simulink model "war_pocz"  (R2014a)
settings: Solver=ode45  StartTime=0.0  StopTime=1  MaxStep=0.5  RelTol=1e-3
values from neighbouring files (symbols this model uses):
  A = [-Kcg1-Kcs-Kcw1 Kcg1 Kcs 0 0 0 ... (first row only)    [blok.m]
  B = [Kcw1 0 ... (first row only)    [blok.m]
  qk0 = x(6,1)    [blok.m]    (also in dom.m = 10000)
  TkpN = 70    [blok.m]    (also in dom.m)
  TkzN = 90    [blok.m]    (also in dom.m)
  Tzew0 = TzewN    (= -20)    [blok.m]    (also in dom.m)
undefined symbols (not defined in the file or in its folder): C, D, Twew1, Twew2
settings Model: Creator=Adrian  LastModifiedBy=Adrian

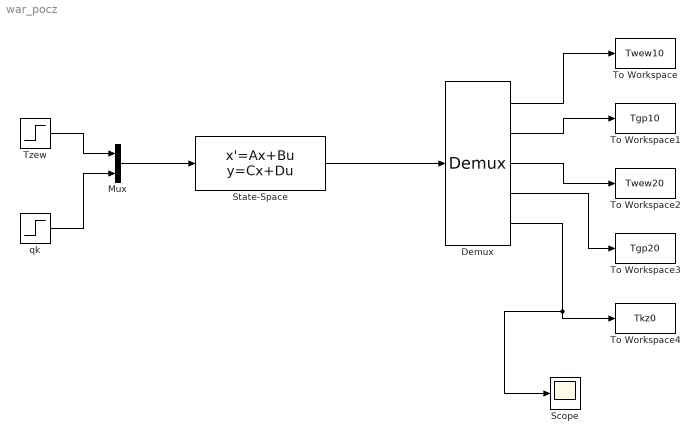
== system war_pocz ==
  Demux : Demux  Outputs=5
  Mux : Mux  Inputs=2
  Scope : Scope
  State-Space : StateSpace  A=A  B=B  C=C  D=D  X0=[Twew1 TkpN Twew2 TkpN TkzN]
  To Workspace : ToWorkspace  VariableName=Twew10  SampleTime=-1
  To Workspace1 : ToWorkspace  VariableName=Tgp10  SampleTime=-1
  To Workspace2 : ToWorkspace  VariableName=Twew20  SampleTime=-1
  To Workspace3 : ToWorkspace  VariableName=Tgp20  SampleTime=-1
  To Workspace4 : ToWorkspace  VariableName=Tkz0  SampleTime=-1
  Tzew : Step  Before=Tzew0  After=Tzew0  SampleTime=0
  qk : Step  Before=qk0  After=qk0  SampleTime=0
  wires:
  Mux/1 -> State-Space/1
  State-Space/1 -> Demux/1
  Tzew/1 -> Mux/1
  qk/1 -> Mux/2
  Demux/5 -> Scope/1, To Workspace4/1
  Demux/4 -> To Workspace3/1
  Demux/3 -> To Workspace2/1
  Demux/2 -> To Workspace1/1
  Demux/1 -> To Workspace/1
